simulink model "model"  (Simulink 7.1)
settings: Solver=ode5  StartTime=0.0  StopTime=50  FixedStep=0.001  RelTol=1e-3
InitFcn:
  | init_para
undefined symbols (not defined in the file): a, dzcv, fc, fp, fs, g, j, l, M, mi, xc, yc
settings Model: Creator=AF1  LastModifiedBy=hussam
settings DataIOCC: SignalLoggingName=sigsOut
settings OptimizationCC: BooleanDataType=off
settings DebuggingCC: SaveWithParameterizedLinksMsg=none  SignalResolutionControl=TryResolveAllWithWarning  SolverPrmCheckMsg=none  MultiTaskDSMMsg=warning  MultiTaskCondExecSysMsg=none  StrictBusMsg=None
settings HardwareCC: TargetUnknown=on
settings RTWCC: IncludeERTFirstTime=on
settings GRTTargetCC: TargetFcnLib=ansi_tfl_tmw.mat

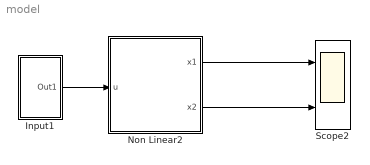
== system model ==
  Input1 : Subsystem
  Non Linear2 : Subsystem
  Scope2 : Scope  NumInputPorts=2
      settings: TimeRange=50  YMin=0~0  YMax=0.35~6  SaveName=ScopeData2
  wires:
  Input1/1(Out1) -> Non Linear2/1(u)
  Non Linear2/1(x1) -> Scope2/1
  Non Linear2/2(x2) -> Scope2/2

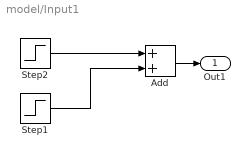
== system model/Input1 ==
  Add : Sum  OutDataType=sfix(16)  OutScaling=2^-10
  Step1 : Step  Time=1.2  After=-.6  SampleTime=0
  Step2 : Step  After=.6  SampleTime=0
  Out1 : Outport  OutDataType=sfix(16)  OutScaling=2^0
  wires:
  Add/1 -> Out1/1
  Step1/1 -> Add/2
  Step2/1 -> Add/1

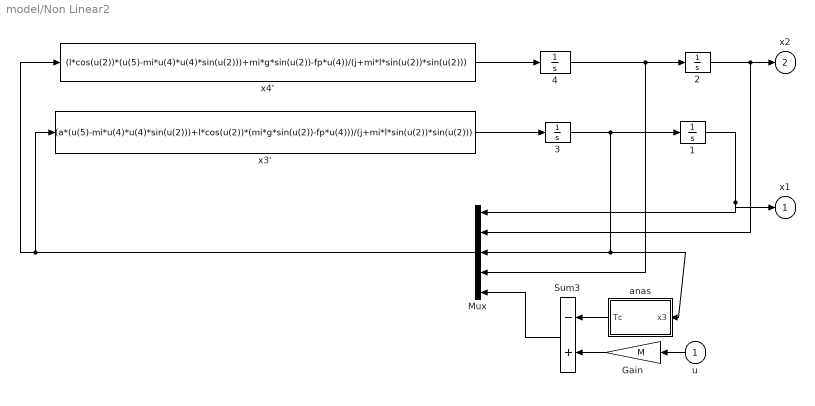
== system model/Non Linear2 ==
  u : Inport  Orientation=left  OutDataType=sfix(16)  OutScaling=2^0
  {1..4} (4 alike) : Integrator
  Gain : Gain  Orientation=left  Gain=M  ParameterDataType=sfix(16)  ParameterScaling=2^0  OutDataType=sfix(16)  OutScaling=2^0  SaturateOnIntegerOverflow=on  OutDataTypeStr=Inherit: Same as input  ParamDataTypeStr=Inherit: Same as input
  Mux : Mux  Orientation=left  Inputs=5
  Sum3 : Sum  Orientation=left  Inputs=-+  OutDataType=sfix(16)  OutScaling=2^0  SaturateOnIntegerOverflow=on
  anas : Subsystem  Orientation=left
  x3' : Fcn  Expr=(a*(u(5)-mi*u(4)*u(4)*sin(u(2)))+l*cos(u(2))*(mi*g*sin(u(2))-fp*u(4)))/(j+mi*l*sin(u(2))*sin(u(2)))
  x4' : Fcn  Expr=(l*cos(u(2))*(u(5)-mi*u(4)*u(4)*sin(u(2)))+mi*g*sin(u(2))-fp*u(4))/(j+mi*l*sin(u(2))*sin(u(2)))
  x1 : Outport  OutDataType=sfix(16)  OutScaling=2^0
  x2 : Outport  Port=2  OutDataType=sfix(16)  OutScaling=2^0
  wires:
  x3'/1 -> 3/1
  x4'/1 -> 4/1
  Sum3/1 -> Mux/5
  anas/1(Tc) -> Sum3/1
  Gain/1 -> Sum3/2
  2/1 -> x2/1, Mux/2
  3/1 -> anas/1(x3), Mux/3, 1/1
  u/1 -> Gain/1
  Mux/1 -> x3'/1, x4'/1
  1/1 -> x1/1, Mux/1
  4/1 -> Mux/4, 2/1

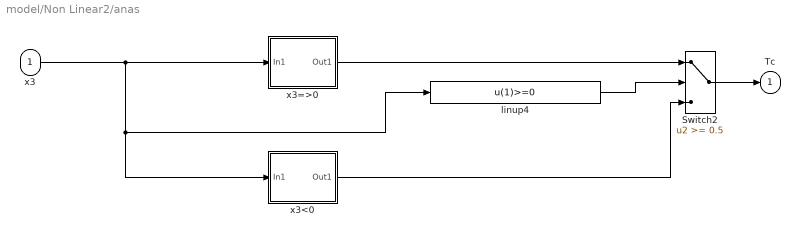
== system model/Non Linear2/anas ==
  x3 : Inport  OutDataType=sfix(16)  OutScaling=2^0
  Switch2 : Switch  Threshold=0.5  SaturateOnIntegerOverflow=on
  linup4 : Fcn  Expr=u(1)>=0
  x3<0 : Subsystem
  x3=>0 : Subsystem
  Tc : Outport
  wires:
  linup4/1 -> Switch2/2
  Switch2/1 -> Tc/1
  x3<0/1(Out1) -> Switch2/3
  x3/1 -> linup4/1, x3<0/1(In1), x3=>0/1(In1)
  x3=>0/1(Out1) -> Switch2/1

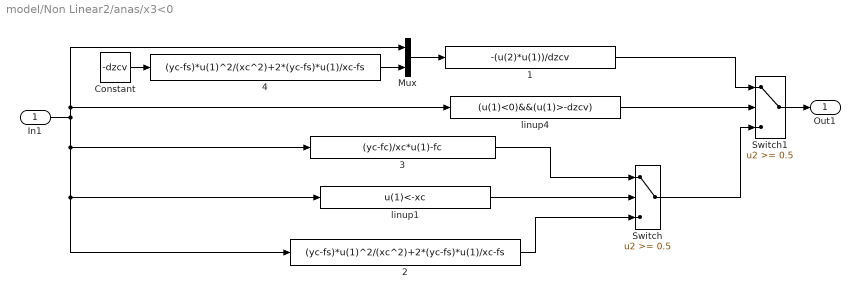
== system model/Non Linear2/anas/x3<0 ==
  In1 : Inport  OutDataType=sfix(16)  OutScaling=2^0
  1 : Fcn  Expr=-(u(2)*u(1))/dzcv
  2 : Fcn  Expr=(yc-fs)*u(1)^2/(xc^2)+2*(yc-fs)*u(1)/xc-fs
  3 : Fcn  Expr=(yc-fc)/xc*u(1)-fc
  4 : Fcn  Expr=(yc-fs)*u(1)^2/(xc^2)+2*(yc-fs)*u(1)/xc-fs
  Constant : Constant  Value=-dzcv  OutDataType=sfix(16)  OutScaling=2^0
  Mux : Mux  Inputs=2
  Switch : Switch  Threshold=0.5  SaturateOnIntegerOverflow=on
  Switch1 : Switch  Threshold=0.5  SaturateOnIntegerOverflow=on
  linup1 : Fcn  Expr=u(1)<-xc
  linup4 : Fcn  Expr=(u(1)<0)&&(u(1)>-dzcv)
  Out1 : Outport  OutDataType=sfix(16)  OutScaling=2^0
  wires:
  Constant/1 -> 4/1
  4/1 -> Mux/2
  Mux/1 -> 1/1
  3/1 -> Switch/1
  2/1 -> Switch/3
  1/1 -> Switch1/1
  linup4/1 -> Switch1/2
  linup1/1 -> Switch/2
  Switch/1 -> Switch1/3
  In1/1 -> Mux/1, linup4/1, 3/1, linup1/1, 2/1
  Switch1/1 -> Out1/1

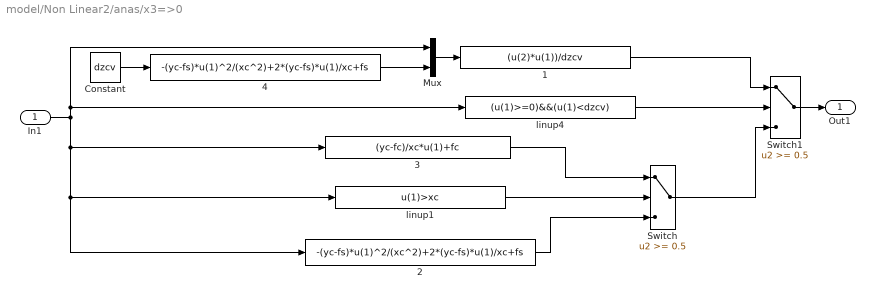
== system model/Non Linear2/anas/x3=>0 ==
  In1 : Inport  OutDataType=sfix(16)  OutScaling=2^0
  1 : Fcn  Expr=(u(2)*u(1))/dzcv
  2 : Fcn  Expr=-(yc-fs)*u(1)^2/(xc^2)+2*(yc-fs)*u(1)/xc+fs
  3 : Fcn  Expr=(yc-fc)/xc*u(1)+fc
  4 : Fcn  Expr=-(yc-fs)*u(1)^2/(xc^2)+2*(yc-fs)*u(1)/xc+fs
  Constant : Constant  Value=dzcv  OutDataType=sfix(16)  OutScaling=2^0
  Mux : Mux  Inputs=2
  Switch : Switch  Threshold=0.5  SaturateOnIntegerOverflow=on
  Switch1 : Switch  Threshold=0.5  SaturateOnIntegerOverflow=on
  linup1 : Fcn  Expr=u(1)>xc
  linup4 : Fcn  Expr=(u(1)>=0)&&(u(1)<dzcv)
  Out1 : Outport  OutDataType=sfix(16)  OutScaling=2^0
  wires:
  Constant/1 -> 4/1
  4/1 -> Mux/2
  Mux/1 -> 1/1
  Switch1/1 -> Out1/1
  In1/1 -> Mux/1, linup4/1, 2/1, linup1/1, 3/1
  Switch/1 -> Switch1/3
  linup1/1 -> Switch/2
  linup4/1 -> Switch1/2
  1/1 -> Switch1/1
  2/1 -> Switch/3
  3/1 -> Switch/1
